simulink model "Python_Testing_Platform_2a"  (R2020b)
settings: Solver=VariableStepAuto  StartTime=0.0  StopTime=10.0  RelTol=1e-3
InitFcn:
  | close all
  | clear
  | clc
  | 
  | dtsim = 0.1;
  | dt =0.005;
  | dtdata = 0.01;
  | dtcontrol = 0.01;
  | 
  | % Enviromental Constants/System Parameters
  | 
  | mu = 398600; %km^3/s^2 (Earth)
  | 
  | I = [1.01560749 0.00028915 0.00002257;
  |        0.00028915 0.17343628 0.00936307;
  |        0.00002257 0.00936307 1.01561864];
  | 
  | I_inv =[1/I(1,1) 0 0; 0 1/I(2,2) 0; 0 0 1/I(3,3)];
  | 
  | % Inital Conditions
  | 
  | Y = 0;
  | P = 0;
  | R = 0;
  | 
  | a = 6378;
  | n = sqrt(mu/a^3);
  | 
  | wo = [0;0;0];
  | ho = [0;0;0];
  | 
  | % YPR to Quaternion
  | 
  | qo = [-cos(R/2)*sin(P/2)*sin(Y/2) + sin(R/2)*cos(P/2)*cos(Y/2);
  |           cos(R/2)*sin(P/2)*cos(Y/2) + sin(R/2)*cos(P/2)*sin(Y/2);
  |          -sin(R/2)*sin(P/2)*cos(Y/2) + cos(R/2)*cos(P/2)*sin(Y/2);
  |           sin(R/2)*sin(P/2)*sin(Y/2) + cos(R/2)*cos(P/2)*cos(Y/2)];
  | 
  | % Reaction Wheels
  | 
  | largeAngle = cosd(70);
  | smallAngle = sind(70);
  | e1 = [largeAngle; smallAngle; 0];
  | e2 = [largeAngle; 0; smallAngle];
  | e3 = [largeAngle; -smallAngle; 0];
  | e4 = [largeAngle; 0; -smallAngle];
  | e = [e1 e2 e3 e4];
  | 
  | % Reaction Wheels MOI and Ang Vel
  | 
  | Irw = 0.000453158;
  | 
  | w1 =1500*2*pi/60;
  | w2 = 1500*2*pi/60;
  | w3 = -1500*2*pi/60;
  | w4 = -1500*2*pi/60;
  | 
  | alpha_max = 1537.9; %rad/sec^2 Look at picture
  | 
  | Tmax = Irw*alpha_max; % Irw*alpha_max;
  | 
  | %User Input
  | 
  | Yt = 90*pi/180;
  | Pt = 10*pi/180;
  | Rt = 30*pi/180;
  | 
  | YPRtarget = [Yt, Pt, Rt];
  | 
  | %User Input Check
  | 
  | if Pt > 20*pi/180
  | 
  | error('Input a pitch angle lower that 20 degrees')
  | 
  | end
  | 
  | q_target = [-cos(Rt/2)*sin(Pt/2)*sin(Yt/2) + sin(Rt/2)*cos(Pt/2)*cos(Yt/2);
  |                   cos(Rt/2)*sin(Pt/2)*cos(Yt/2) + sin(Rt/2)*cos(Pt/2)*sin(Yt/2);
  |                  -sin(Rt/2)*sin(Pt/2)*cos(Yt/2) + cos(Rt/2)*cos(Pt/2)*sin(Yt/2);
  |                   sin(Rt/2)*sin(Pt/2)*sin(Yt/2) + cos(Rt/2)*cos(Pt/2)*cos(Yt/2)];
  | 
  | %LQR Controller
  | 
  | k1 = (I(2,2) - I(3,3))/I(1,1);
  | k2 = (I(2,2) - I(3,3))/I(2,2);
  | k3 = (I(2,2) - I(1,1))/I(3,3);
  | 
  | F = -2*n^2*[4*k1, 0, 0;0, 3*k2, 0; 0, 0, k3];
  | G = n*[0 0 (1-k1);0 0 0;(k3-1) 0 0 ];
  | 
  | A = [zeros(3,3) 0.5*eye(3);F G];
  | B = [zeros(3,3); I_inv];
  | R = eye(3);
  | R_inv = R^-1;
  | 
  | Q_nominal= diag([1,1,1,10,10,10]);
  | S_nominal = icare(A,B,Q_nominal,R);
  | K_nominal = -R_inv*B'*S_nominal;
  | 
  | Q_corrective= diag([1,1,1,10,10,10]);
  | S_corrective = icare(A,B,Q_corrective,R);
  | K_corrective = -R_inv*B'*S_corrective;
  | 
  | Q_yawsweep= diag([1,1,1,10,15,10]);
  | S_yawsweep = icare(A,B,Q_yawsweep,R);
  | K_yawsweep = -R_inv*B'*S_yawsweep;
libraries: dspinverses x1
settings Model: Creator=Eric Malmquist  LastModifiedBy=Eric Malmquist

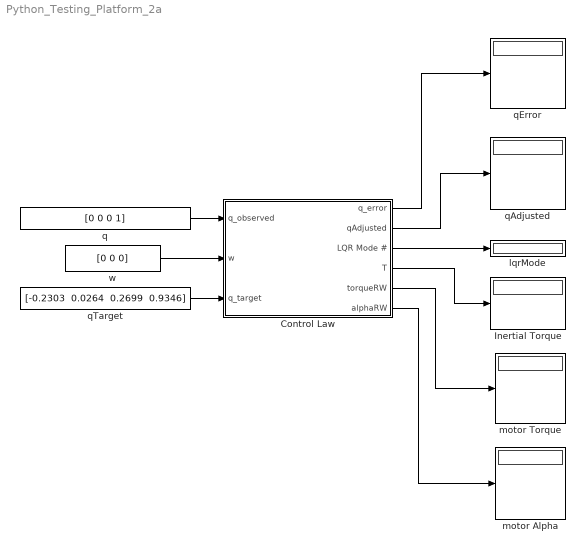
== system Python_Testing_Platform_2a ==
  Control Law : Subsystem
  Inertial Torque : Display
  lqrMode : Display
  motor Alpha : Display
  motor Torque : Display
  q : Constant  Value=[0 0 0 1]
  qAdjusted : Display
  qError : Display
  qTarget : Constant  Value="[-0.2303  0.0264  0.2699  0.9346]"
  w : Constant  Value=[0 0 0]
  wires:
  Control Law/4(T) -> Inertial Torque/1
  Control Law/2(qAdjusted) -> qAdjusted/1
  Control Law/3(LQR Mode #) -> lqrMode/1
  qTarget/1 -> Control Law/3(q_target)
  w/1 -> Control Law/2(w)
  Control Law/1(q_error) -> qError/1
  Control Law/5(torqueRW) -> motor Torque/1
  Control Law/6(alphaRW) -> motor Alpha/1
  q/1 -> Control Law/1(q_observed)

== system Python_Testing_Platform_2a/Control Law ==
  q_observed : Inport
  w : Inport  Port=2
  q_target : Inport  Port=3
  Controller1 : Subsystem
  Motor Control1 : Subsystem
  qerror1 : Subsystem
  q_error : Outport
  qAdjusted : Outport  Port=2
  LQR Mode # : Outport  Port=3
  T : Outport  Port=4
  torqueRW : Outport  Port=5
  alphaRW : Outport  Port=6
  wires:
  qerror1/3(Roll_ErrorAbs) -> Controller1/3(Roll_ErrorAbs)
  q_target/1 -> qerror1/1(q_target), Controller1/6(target)
  Controller1/3(Out1) -> LQR Mode #/1
  q_observed/1 -> qerror1/2(q_observed), Controller1/4(q_obs)
  Controller1/1(T) -> T/1, Motor Control1/1(T)
  qerror1/2(Yaw_ErrorAbs) -> Controller1/2(Yaw_ErrorAbs)
  qerror1/1(q_error) -> q_error/1, Controller1/1(q_error)
  w/1 -> Controller1/5(w)
  Motor Control1/1(torqueRW) -> torqueRW/1
  Motor Control1/2(alphaRW) -> alphaRW/1
  Controller1/2(qAdjusted) -> qAdjusted/1

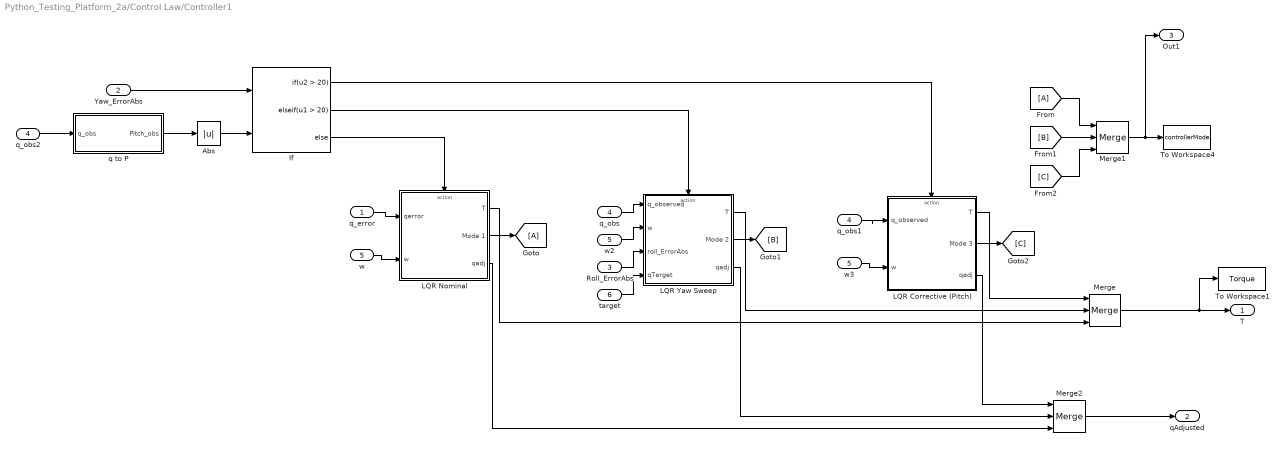
== system Python_Testing_Platform_2a/Control Law/Controller1 ==
  q_error : Inport
  Yaw_ErrorAbs : Inport  Port=2
  Roll_ErrorAbs : Inport  Port=3
  q_obs : Inport  Port=4
  w : Inport  Port=5
  target : Inport  Port=6
  Abs : Abs
  If : If  NumInputs=2  IfExpression=u2 > 20  ElseIfExpressions=u1 > 20
  LQR Corrective (Pitch) : Subsystem
  LQR Nominal : Subsystem  TreatAsAtomicUnit=on
  LQR Yaw Sweep : Subsystem
  Merge : Merge  Inputs=3
  Merge1 : Merge  Inputs=3
  Merge2 : Merge  Inputs=3
  To Workspace1 : ToWorkspace  VariableName=Torque  SaveFormat=Structure With Time  SampleTime=-1
  To Workspace4 : ToWorkspace  VariableName=controllerMode  SaveFormat=Structure With Time  SampleTime=-1
  q to P : Subsystem
  q_obs1 : InportShadow  Port=4
  q_obs2 : InportShadow  Port=4
  w2 : InportShadow  Port=5
  w3 : InportShadow  Port=5
  T : Outport
  qAdjusted : Outport  Port=2
  Out1 : Outport  Port=3
  wires:
  Yaw_ErrorAbs/1 -> If/1
  If/3 -> LQR Nominal/Action
  q_error/1 -> LQR Nominal/1(qerror)
  If/1 -> LQR Corrective (Pitch)/Action
  q_obs1/1 -> LQR Corrective (Pitch)/1(q_observed)
  q_obs/1 -> LQR Yaw Sweep/1(q_observed)
  q to P/1(Pitch_obs) -> Abs/1
  If/2 -> LQR Yaw Sweep/Action
  LQR Nominal/2(Mode 1) -> [A]
  LQR Yaw Sweep/2(Mode 2) -> [B]
  LQR Corrective (Pitch)/2(Mode 3) -> [C]
  [B] -> Merge1/2
  [A] -> Merge1/1
  [C] -> Merge1/3
  Merge1/1 -> Out1/1, To Workspace4/1
  w3/1 -> LQR Corrective (Pitch)/2(w)
  w2/1 -> LQR Yaw Sweep/2(w)
  w/1 -> LQR Nominal/2(w)
  q_obs2/1 -> q to P/1(q_obs)
  Abs/1 -> If/2
  Roll_ErrorAbs/1 -> LQR Yaw Sweep/3(roll_ErrorAbs)
  LQR Nominal/1(T) -> Merge/3
  LQR Yaw Sweep/1(T) -> Merge/2
  LQR Corrective (Pitch)/1(T) -> Merge/1
  Merge/1 -> To Workspace1/1, T/1
  LQR Nominal/3(qadj) -> Merge2/3
  LQR Yaw Sweep/3(qadj) -> Merge2/2
  LQR Corrective (Pitch)/3(qadj) -> Merge2/1
  Merge2/1 -> qAdjusted/1
  target/1 -> LQR Yaw Sweep/4(qTarget)

== system Python_Testing_Platform_2a/Control Law/Motor Control1 ==
  T : Inport
  Actuator : Subsystem
  torqueRW : Outport
  alphaRW : Outport  Port=2
  wires:
  T/1 -> Actuator/1(Torque)
  Actuator/2(torque) -> torqueRW/1
  Actuator/1(alpha_RW) -> alphaRW/1

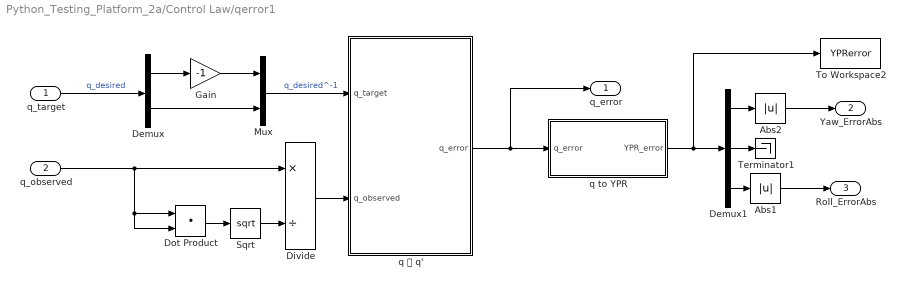
== system Python_Testing_Platform_2a/Control Law/qerror1 ==
  q_target : Inport
  q_observed : Inport  Port=2
  Abs1 : Abs
  Abs2 : Abs
  Demux : Demux  Outputs=[3,1]
  Demux1 : Demux  Outputs=3
  Divide : Product  Inputs=*/
  Dot Product : DotProduct  InputSameDT=on  OutDataTypeStr=Inherit: Inherit via internal rule
  Gain : Gain  Gain=-1
  Mux : Mux  Inputs=2
  Sqrt : Sqrt  SaturateOnIntegerOverflow=on
  Terminator1 : Terminator
  To Workspace2 : ToWorkspace  VariableName=YPRerror  SaveFormat=Structure With Time  SampleTime=-1
  q to YPR : Subsystem  TreatAsAtomicUnit=on
  q ⦻ q' : Subsystem  TreatAsAtomicUnit=on
  q_error : Outport
  Yaw_ErrorAbs : Outport  Port=2
  Roll_ErrorAbs : Outport  Port=3
  wires:
  Abs2/1 -> Yaw_ErrorAbs/1
  Demux1/2 -> Terminator1/1
  Abs1/1 -> Roll_ErrorAbs/1
  Divide/1 -> q ⦻ q'/2(q_observed)
  q_observed/1 -> Divide/1, Dot Product/1, Dot Product/2
  Dot Product/1 -> Sqrt/1
  q ⦻ q'/1(q_error) -> q to YPR/1(q_error), q_error/1
  Gain/1 -> Mux/1
  Mux/1 -> q ⦻ q'/1(q_target)  "q_desired^-1"
  q_target/1 -> Demux/1  "q_desired"
  Demux/1 -> Gain/1
  Sqrt/1 -> Divide/2
  Demux/2 -> Mux/2
  q to YPR/1(YPR_error) -> Demux1/1, To Workspace2/1
  Demux1/1 -> Abs2/1
  Demux1/3 -> Abs1/1

== system Python_Testing_Platform_2a/Control Law/Controller1/LQR Corrective (Pitch) ==
  q_observed : Inport
  w : Inport  Port=2
  Action Port : ActionPort  ActionPortLabel=if(u2 > 20)
  Constant : Constant  Value=3
  LQR Corrective (Pitch) : Subsystem
  q_adjustment : Subsystem
  q_error : Subsystem
  T : Outport
  Mode 3 : Outport  Port=2
  qadj : Outport  Port=3
  wires:
  Constant/1 -> Mode 3/1
  LQR Corrective (Pitch)/1(T) -> T/1
  w/1 -> LQR Corrective (Pitch)/2(w)
  q_adjustment/1(q_adjusted) -> q_error/1(q_target)
  q_observed/1 -> q_adjustment/1(q_obs), q_error/2(q_observed)
  q_error/1(q_error) -> qadj/1, LQR Corrective (Pitch)/1(q_error)

== system Python_Testing_Platform_2a/Control Law/Controller1/LQR Nominal ==
  qerror : Inport
  w : Inport  Port=2
  Action Port : ActionPort  ActionPortLabel=else
  Constant : Constant
  LQR Nominal : Subsystem
  T : Outport
  Mode 1 : Outport  Port=2
  qadj : Outport  Port=3
  wires:
  Constant/1 -> Mode 1/1
  LQR Nominal/1(T) -> T/1
  w/1 -> LQR Nominal/2(w)
  qerror/1 -> qadj/1, LQR Nominal/1(q_error)

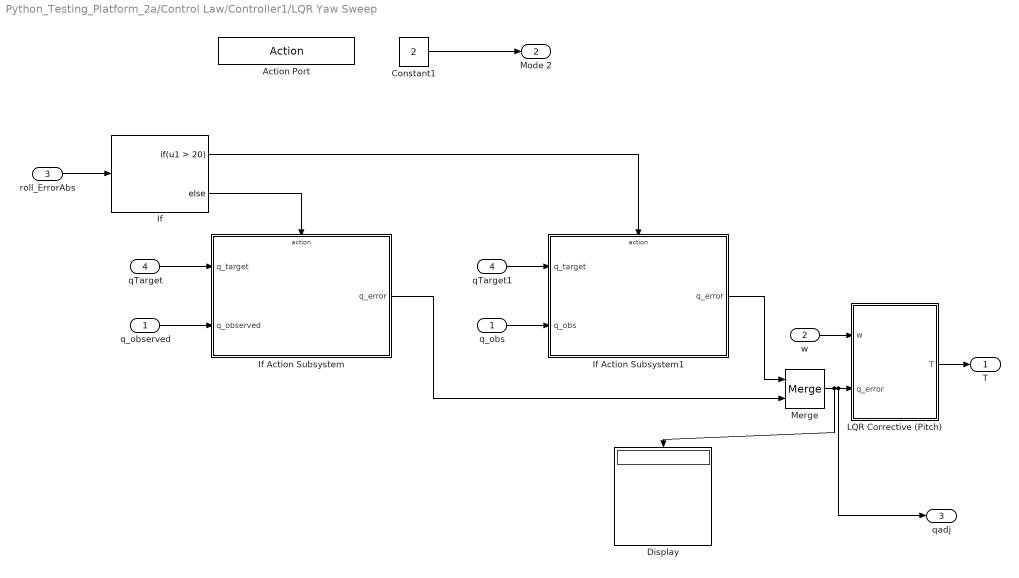
== system Python_Testing_Platform_2a/Control Law/Controller1/LQR Yaw Sweep ==
  q_observed : Inport
  w : Inport  Port=2
  roll_ErrorAbs : Inport  Port=3
  qTarget : Inport  Port=4
  Action Port : ActionPort  ActionPortLabel=elseif(u1 > 20)
  Constant1 : Constant  Value=2
  Display : Display
  If : If  IfExpression=u1 > 20
  If Action Subsystem : Subsystem  TreatAsAtomicUnit=on
  If Action Subsystem1 : Subsystem  TreatAsAtomicUnit=on
  LQR Corrective (Pitch) : Subsystem
  Merge : Merge
  qTarget1 : InportShadow  Port=4
  q_obs : InportShadow
  T : Outport
  Mode 2 : Outport  Port=2
  qadj : Outport  Port=3
  wires:
  roll_ErrorAbs/1 -> If/1
  qTarget/1 -> If Action Subsystem/1(q_target)
  Constant1/1 -> Mode 2/1
  If/2 -> If Action Subsystem/Action
  LQR Corrective (Pitch)/1(T) -> T/1
  w/1 -> LQR Corrective (Pitch)/1(w)
  If/1 -> If Action Subsystem1/Action
  q_observed/1 -> If Action Subsystem/2(q_observed)
  Merge/1 -> Display/1, qadj/1, LQR Corrective (Pitch)/2(q_error)
  If Action Subsystem1/1(q_error) -> Merge/1
  If Action Subsystem/1(q_error) -> Merge/2
  q_obs/1 -> If Action Subsystem1/2(q_obs)
  qTarget1/1 -> If Action Subsystem1/1(q_target)

== system Python_Testing_Platform_2a/Control Law/Controller1/q to P ==
  q_obs : Inport
  -DCM(1,3) : Fcn  Expr=-2*(u(1)*u(3) - u(2)*u(4))
  Gain2 : Gain  Gain=180/pi
  Trigonometric Function1 : Trigonometry  Operator=asin
  Pitch_obs : Outport
  wires:
  Gain2/1 -> Pitch_obs/1
  Trigonometric Function1/1 -> Gain2/1  "P"
  -DCM(1,3)/1 -> Trigonometric Function1/1
  q_obs/1 -> -DCM(1,3)/1

== system Python_Testing_Platform_2a/Control Law/Motor Control1/Actuator ==
  Torque : Inport  PortDimensions=[3,1]
  Constant1 : Constant  Value=Irw
  Constant2 : Constant  Value=e
  Constant3 : Constant  Value=Irw
  Gain : Gain  Gain=-1
  Multiply : Product  Multiplication=Matrix(*)
  Product : Product
  Product1 : Product
  Pseudoinverse : dspinverses/Pseudoinverse  wanterr=off  SimulateUsing=Interpreted execution
      settings: SourceProductBaseCode=DS
  Rate Transition1 : RateTransition  InitialCondition=[0;0;0;0]  OutPortSampleTime=dtdata
  alpha_RW : Outport
  torque : Outport  Port=2
  wires:
  Torque/1 -> Gain/1
  Product/1 -> Pseudoinverse/1
  Constant1/1 -> Product/1
  Pseudoinverse/1 -> Multiply/1  "psiv(A)"
  Multiply/1 -> Product1/1, alpha_RW/1  "alpha_RW"
  Constant2/1 -> Product/2  "A"
  Gain/1 -> Multiply/2
  Constant3/1 -> Product1/2
  Product1/1 -> Rate Transition1/1
  Rate Transition1/1 -> torque/1

== system Python_Testing_Platform_2a/Control Law/qerror1/q to YPR ==
  note: Quaternion to Euler Angles using sequency 3-2-1
  q_error : Inport
  -DCM(1,3) : Fcn  Expr=-2*(u(1)*u(3) - u(2)*u(4))
  DCM(1,1) : Fcn  Expr=u(4)^2 + u(1)^2 - u(2)^2 - u(3)^2
  DCM(1,2) : Fcn  Expr=2*(u(1)*u(2) + u(3)*u(4))
  DCM(2,3) : Fcn  Expr=2*(u(2)*u(3) + u(1)*u(4))
  DCM(3,3) : Fcn  Expr=u(4)^2 - u(1)^2 - u(2)^2 + u(3)^2
  Gain2 : Gain  Gain=180/pi
  Mux : Mux  Inputs=3
  Trigonometric Function : Trigonometry  Operator=asin
  Trigonometric Function1 : Trigonometry  Operator=atan2
  Trigonometric Function2 : Trigonometry  Operator=atan2
  YPR_error : Outport
  wires:
  q_error/1 -> DCM(3,3)/1, DCM(2,3)/1, -DCM(1,3)/1, DCM(1,2)/1, DCM(1,1)/1
  -DCM(1,3)/1 -> Trigonometric Function/1
  DCM(2,3)/1 -> Trigonometric Function2/1
  DCM(1,2)/1 -> Trigonometric Function1/1
  DCM(1,1)/1 -> Trigonometric Function1/2
  DCM(3,3)/1 -> Trigonometric Function2/2
  Trigonometric Function/1 -> Mux/2  "P"
  Trigonometric Function2/1 -> Mux/3  "R"
  Trigonometric Function1/1 -> Mux/1  "Y"
  Gain2/1 -> YPR_error/1
  Mux/1 -> Gain2/1

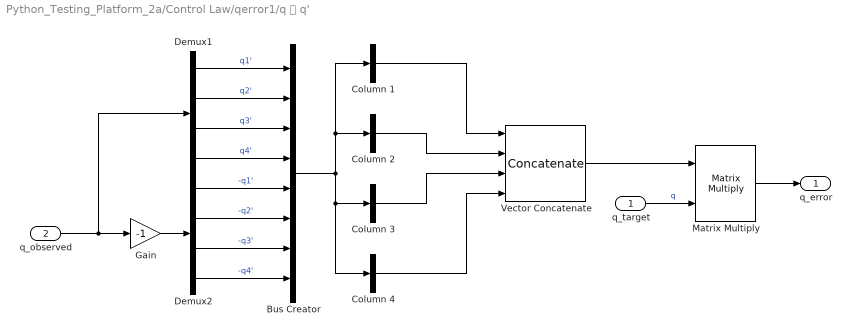
== system Python_Testing_Platform_2a/Control Law/qerror1/q ⦻ q' ==
  q_target : Inport
  q_observed : Inport  Port=2
  Bus Creator : BusCreator  Inputs=8
  Column 1 : BusSelector  OutputSignals=q4',-q3',q2',-q1'  OutputAsBus=on
  Column 2 : BusSelector  OutputSignals=q3',q4',-q1',-q2'  OutputAsBus=on
  Column 3 : BusSelector  OutputSignals=-q2',q1',q4',-q3'  OutputAsBus=on
  Column 4 : BusSelector  OutputSignals=q1',q2',q3',q4'  OutputAsBus=on
  Demux1 : Demux
  Demux2 : Demux
  Gain : Gain  Gain=-1
  Matrix Multiply : Product  Multiplication=Matrix(*)
  Vector Concatenate : Concatenate  NumInputs=4  Mode=Multidimensional array  ConcatenateDimension=2
  q_error : Outport
  wires:
  Gain/1 -> Demux2/1
  Demux1/1 -> Bus Creator/1  "q1'"
  Demux1/3 -> Bus Creator/3  "q3'"
  Demux1/2 -> Bus Creator/2  "q2'"
  Demux2/4 -> Bus Creator/8  "-q4'"
  Demux2/3 -> Bus Creator/7  "-q3'"
  Demux2/2 -> Bus Creator/6  "-q2'"
  Demux2/1 -> Bus Creator/5  "-q1'"
  Demux1/4 -> Bus Creator/4  "q4'"
  Bus Creator/1 -> Column 4/1, Column 3/1, Column 1/1, Column 2/1
  Column 1/1 -> Vector Concatenate/1
  Column 2/1 -> Vector Concatenate/2
  Column 3/1 -> Vector Concatenate/3
  Column 4/1 -> Vector Concatenate/4
  q_observed/1 -> Demux1/1, Gain/1
  q_target/1 -> Matrix Multiply/2  "q"
  Matrix Multiply/1 -> q_error/1
  Vector Concatenate/1 -> Matrix Multiply/1

== system Python_Testing_Platform_2a/Control Law/Controller1/LQR Corrective (Pitch)/LQR Corrective (Pitch) ==
  q_error : Inport
  w : Inport  Port=2
  Constant3 : Constant  Value=K_corrective
  Demux1 : Demux  Outputs=[3,1]
  Mux1 : Mux  Inputs=2
  Product : Product  Multiplication=Matrix(*)
  Terminator1 : Terminator
  T : Outport
  wires:
  Product/1 -> T/1
  q_error/1 -> Demux1/1
  Constant3/1 -> Product/1
  Demux1/1 -> Mux1/1  "qhat_Error"
  w/1 -> Mux1/2
  Mux1/1 -> Product/2  "xbar"
  Demux1/2 -> Terminator1/1

== system Python_Testing_Platform_2a/Control Law/Controller1/LQR Corrective (Pitch)/q_adjustment ==
  q_obs : Inport
  DCM(1,1) : Fcn  Expr=u(4)^2 + u(1)^2 - u(2)^2 - u(3)^2
  DCM(1,2) : Fcn  Expr=2*(u(1)*u(2) + u(3)*u(4))
  DCM(2,3) : Fcn  Expr=2*(u(2)*u(3) + u(1)*u(4))
  DCM(3,3) : Fcn  Expr=u(4)^2 - u(1)^2 - u(2)^2 + u(3)^2
  Trigonometric Function4 : Trigonometry  Operator=atan2
  Trigonometric Function5 : Trigonometry  Operator=atan2
  YPR to q : Subsystem
  q_adjusted : Outport
  wires:
  Trigonometric Function5/1 -> YPR to q/2(R)  "R"
  DCM(2,3)/1 -> Trigonometric Function5/1
  DCM(1,1)/1 -> Trigonometric Function4/2
  DCM(3,3)/1 -> Trigonometric Function5/2
  DCM(1,2)/1 -> Trigonometric Function4/1
  q_obs/1 -> DCM(3,3)/1, DCM(2,3)/1, DCM(1,2)/1, DCM(1,1)/1
  YPR to q/1(q_adjusted) -> q_adjusted/1
  Trigonometric Function4/1 -> YPR to q/1(Y)  "Y"

== system Python_Testing_Platform_2a/Control Law/Controller1/LQR Corrective (Pitch)/q_error ==
  q_target : Inport
  q_observed : Inport  Port=2
  Demux : Demux  Outputs=[3,1]
  Divide : Product  Inputs=*/
  Dot Product : DotProduct  InputSameDT=on  OutDataTypeStr=Inherit: Inherit via internal rule
  Gain : Gain  Gain=-1
  Mux : Mux  Inputs=2
  Sqrt : Sqrt  SaturateOnIntegerOverflow=on
  q ⦻ q' : Subsystem  TreatAsAtomicUnit=on
  q_error : Outport
  wires:
  q ⦻ q'/1(q_error) -> q_error/1
  Mux/1 -> q ⦻ q'/1(q_target)  "q_desired^-1"
  Sqrt/1 -> Divide/2
  Demux/1 -> Gain/1
  q_target/1 -> Demux/1  "q_desired"
  Gain/1 -> Mux/1
  q_observed/1 -> Divide/1, Dot Product/1, Dot Product/2
  Dot Product/1 -> Sqrt/1
  Demux/2 -> Mux/2
  Divide/1 -> q ⦻ q'/2(q_observed)

== system Python_Testing_Platform_2a/Control Law/Controller1/LQR Nominal/LQR Nominal ==
  q_error : Inport
  w : Inport  Port=2
  Constant3 : Constant  Value=K_nominal
  Demux1 : Demux  Outputs=[3,1]
  Mux1 : Mux  Inputs=2
  Product : Product  Multiplication=Matrix(*)
  Terminator1 : Terminator
  T : Outport
  wires:
  Mux1/1 -> Product/2  "xbar"
  Demux1/1 -> Mux1/1  "qhat_Error"
  q_error/1 -> Demux1/1
  Demux1/2 -> Terminator1/1
  w/1 -> Mux1/2
  Constant3/1 -> Product/1
  Product/1 -> T/1

== system Python_Testing_Platform_2a/Control Law/Controller1/LQR Yaw Sweep/If Action Subsystem ==
  q_target : Inport
  q_observed : Inport  Port=2
  Action Port : ActionPort  ActionPortLabel=else
  Display : Display
  Display1 : Display
  Display2 : Display
  q_adjustment : Subsystem
  qerror : Subsystem
  q_error : Outport
  wires:
  q_target/1 -> q_adjustment/1(q_target), Display2/1
  qerror/1(q_error) -> Display1/1, q_error/1
  q_observed/1 -> Display/1, qerror/2(q_observed)
  q_adjustment/1(q_adjusted) -> qerror/1(q_target)

== system Python_Testing_Platform_2a/Control Law/Controller1/LQR Yaw Sweep/If Action Subsystem1 ==
  q_target : Inport
  q_obs : Inport  Port=2
  Action Port : ActionPort  ActionPortLabel=if(u1 > 20)
  q_adjustment : Subsystem
  qerror : Subsystem
  q_error : Outport
  wires:
  q_adjustment/1(q_adjusted) -> qerror/1(q_target)
  q_target/1 -> q_adjustment/1(q_target)
  q_obs/1 -> qerror/2(q_observed), q_adjustment/2(q_obs)
  qerror/1(q_error) -> q_error/1

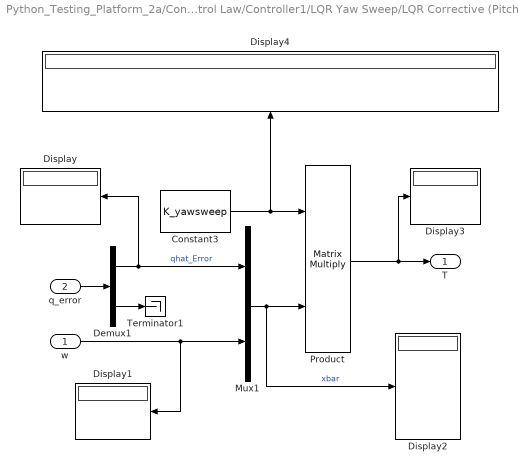
== system Python_Testing_Platform_2a/Control Law/Controller1/LQR Yaw Sweep/LQR Corrective (Pitch) ==
  w : Inport
  q_error : Inport  Port=2
  Constant3 : Constant  Value=K_yawsweep
  Demux1 : Demux  Outputs=[3,1]
  Display{,1..4} (5 alike) : Display
  Mux1 : Mux  Inputs=2
  Product : Product  Multiplication=Matrix(*)
  Terminator1 : Terminator
  T : Outport
  wires:
  Product/1 -> Display3/1, T/1
  q_error/1 -> Demux1/1
  Constant3/1 -> Product/1, Display4/1
  Demux1/1 -> Display/1, Mux1/1  "qhat_Error"
  w/1 -> Display1/1, Mux1/2
  Mux1/1 -> Display2/1, Product/2  "xbar"
  Demux1/2 -> Terminator1/1

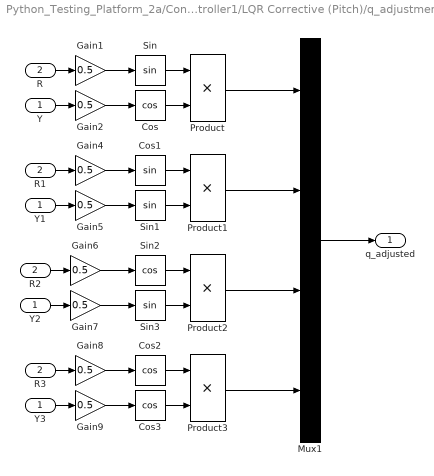
== system Python_Testing_Platform_2a/Control Law/Controller1/LQR Corrective (Pitch)/q_adjustment/YPR to q ==
  Y : Inport
  R : Inport  Port=2
  Cos : Trigonometry  Operator=cos
  Cos1 : Trigonometry
  Cos2 : Trigonometry  Operator=cos
  Cos3 : Trigonometry  Operator=cos
  Gain{1..2,4..9} (8 alike) : Gain  Gain=0.5
  Mux1 : Mux
  Product{,1..3} (4 alike) : Product
  R1 : InportShadow  Port=2
  R2 : InportShadow  Port=2
  R3 : InportShadow  Port=2
  Sin : Trigonometry
  Sin1 : Trigonometry
  Sin2 : Trigonometry  Operator=cos
  Sin3 : Trigonometry
  Y1 : InportShadow
  Y2 : InportShadow
  Y3 : InportShadow
  q_adjusted : Outport
  wires:
  Gain2/1 -> Cos/1
  Sin/1 -> Product/1
  Sin3/1 -> Product2/2
  Sin1/1 -> Product1/2
  Mux1/1 -> q_adjusted/1
  Cos/1 -> Product/2
  Sin2/1 -> Product2/1
  Gain8/1 -> Cos2/1
  Cos1/1 -> Product1/1
  Gain6/1 -> Sin2/1
  Product3/1 -> Mux1/4
  Product/1 -> Mux1/1
  Gain5/1 -> Sin1/1
  Gain9/1 -> Cos3/1
  Gain4/1 -> Cos1/1
  Cos2/1 -> Product3/1
  Product1/1 -> Mux1/2
  Gain7/1 -> Sin3/1
  Gain1/1 -> Sin/1
  Cos3/1 -> Product3/2
  R1/1 -> Gain4/1
  Y1/1 -> Gain5/1
  R2/1 -> Gain6/1
  Y2/1 -> Gain7/1
  Y3/1 -> Gain9/1
  R3/1 -> Gain8/1
  Y/1 -> Gain2/1
  R/1 -> Gain1/1
  Product2/1 -> Mux1/3

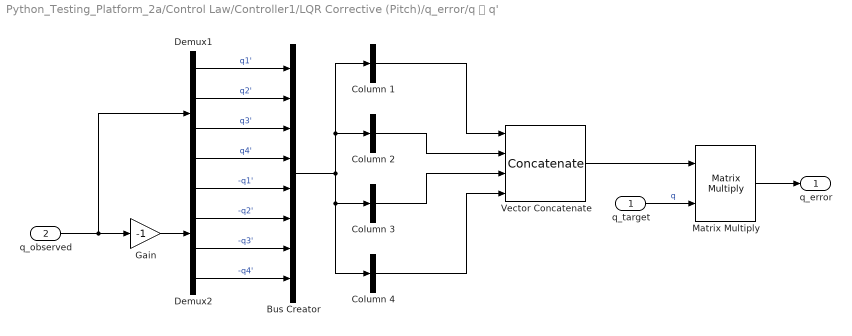
== system Python_Testing_Platform_2a/Control Law/Controller1/LQR Corrective (Pitch)/q_error/q ⦻ q' ==
  q_target : Inport
  q_observed : Inport  Port=2
  Bus Creator : BusCreator  Inputs=8
  Column 1 : BusSelector  OutputSignals=q4',-q3',q2',-q1'  OutputAsBus=on
  Column 2 : BusSelector  OutputSignals=q3',q4',-q1',-q2'  OutputAsBus=on
  Column 3 : BusSelector  OutputSignals=-q2',q1',q4',-q3'  OutputAsBus=on
  Column 4 : BusSelector  OutputSignals=q1',q2',q3',q4'  OutputAsBus=on
  Demux1 : Demux
  Demux2 : Demux
  Gain : Gain  Gain=-1
  Matrix Multiply : Product  Multiplication=Matrix(*)
  Vector Concatenate : Concatenate  NumInputs=4  Mode=Multidimensional array  ConcatenateDimension=2
  q_error : Outport
  wires:
  Gain/1 -> Demux2/1
  Demux1/1 -> Bus Creator/1  "q1'"
  Demux1/3 -> Bus Creator/3  "q3'"
  Demux1/2 -> Bus Creator/2  "q2'"
  Demux2/4 -> Bus Creator/8  "-q4'"
  Demux2/3 -> Bus Creator/7  "-q3'"
  Demux2/2 -> Bus Creator/6  "-q2'"
  Demux2/1 -> Bus Creator/5  "-q1'"
  Demux1/4 -> Bus Creator/4  "q4'"
  Bus Creator/1 -> Column 4/1, Column 3/1, Column 1/1, Column 2/1
  Column 1/1 -> Vector Concatenate/1
  Column 2/1 -> Vector Concatenate/2
  Column 3/1 -> Vector Concatenate/3
  Column 4/1 -> Vector Concatenate/4
  q_observed/1 -> Demux1/1, Gain/1
  q_target/1 -> Matrix Multiply/2  "q"
  Matrix Multiply/1 -> q_error/1
  Vector Concatenate/1 -> Matrix Multiply/1

== system Python_Testing_Platform_2a/Control Law/Controller1/LQR Yaw Sweep/If Action Subsystem/q_adjustment ==
  q_target : Inport
  DCM(1,1) : Fcn  Expr=u(4)^2 + u(1)^2 - u(2)^2 - u(3)^2
  DCM(1,2) : Fcn  Expr=2*(u(1)*u(2) + u(3)*u(4))
  DCM(2,3) : Fcn  Expr=2*(u(2)*u(3) + u(1)*u(4))
  DCM(3,3) : Fcn  Expr=u(4)^2 - u(1)^2 - u(2)^2 + u(3)^2
  Trigonometric Function4 : Trigonometry  Operator=atan2
  Trigonometric Function5 : Trigonometry  Operator=atan2
  YPR to q : Subsystem
  q_adjusted : Outport
  wires:
  YPR to q/1(q_adjusted) -> q_adjusted/1
  Trigonometric Function5/1 -> YPR to q/2(R)  "R"
  DCM(3,3)/1 -> Trigonometric Function5/2
  DCM(1,1)/1 -> Trigonometric Function4/2
  DCM(2,3)/1 -> Trigonometric Function5/1
  Trigonometric Function4/1 -> YPR to q/1(Y)  "Y"
  DCM(1,2)/1 -> Trigonometric Function4/1
  q_target/1 -> DCM(3,3)/1, DCM(2,3)/1, DCM(1,2)/1, DCM(1,1)/1

== system Python_Testing_Platform_2a/Control Law/Controller1/LQR Yaw Sweep/If Action Subsystem/qerror ==
  q_target : Inport
  q_observed : Inport  Port=2
  Demux : Demux  Outputs=[3,1]
  Divide : Product  Inputs=*/
  Dot Product : DotProduct  InputSameDT=on  OutDataTypeStr=Inherit: Inherit via internal rule
  Gain : Gain  Gain=-1
  Mux : Mux  Inputs=2
  Sqrt : Sqrt  SaturateOnIntegerOverflow=on
  q ⦻ q' : Subsystem  TreatAsAtomicUnit=on
  q_error : Outport
  wires:
  Sqrt/1 -> Divide/2
  Dot Product/1 -> Sqrt/1
  Gain/1 -> Mux/1
  Mux/1 -> q ⦻ q'/1(q_target)  "q_desired^-1"
  q ⦻ q'/1(q_error) -> q_error/1
  q_observed/1 -> Divide/1, Dot Product/1, Dot Product/2
  q_target/1 -> Demux/1  "q_desired"
  Demux/1 -> Gain/1
  Demux/2 -> Mux/2
  Divide/1 -> q ⦻ q'/2(q_observed)

== system Python_Testing_Platform_2a/Control Law/Controller1/LQR Yaw Sweep/If Action Subsystem1/q_adjustment ==
  q_target : Inport
  q_obs : Inport  Port=2
  DCM(1,1) : Fcn  Expr=u(4)^2 + u(1)^2 - u(2)^2 - u(3)^2
  DCM(1,2) : Fcn  Expr=2*(u(1)*u(2) + u(3)*u(4))
  DCM(2,3) : Fcn  Expr=2*(u(2)*u(3) + u(1)*u(4))
  DCM(3,3) : Fcn  Expr=u(4)^2 - u(1)^2 - u(2)^2 + u(3)^2
  Trigonometric Function4 : Trigonometry  Operator=atan2
  Trigonometric Function5 : Trigonometry  Operator=atan2
  YPR to q : Subsystem
  q_adjusted : Outport
  wires:
  YPR to q/1(q_adjusted) -> q_adjusted/1
  Trigonometric Function5/1 -> YPR to q/2(R)  "R"
  DCM(1,1)/1 -> Trigonometric Function4/2
  DCM(3,3)/1 -> Trigonometric Function5/2
  DCM(1,2)/1 -> Trigonometric Function4/1
  DCM(2,3)/1 -> Trigonometric Function5/1
  Trigonometric Function4/1 -> YPR to q/1(Y)  "Y"
  q_target/1 -> DCM(1,1)/1, DCM(1,2)/1
  q_obs/1 -> DCM(2,3)/1, DCM(3,3)/1

== system Python_Testing_Platform_2a/Control Law/Controller1/LQR Yaw Sweep/If Action Subsystem1/qerror ==
  q_target : Inport
  q_observed : Inport  Port=2
  Demux : Demux  Outputs=[3,1]
  Divide : Product  Inputs=*/
  Dot Product : DotProduct  InputSameDT=on  OutDataTypeStr=Inherit: Inherit via internal rule
  Gain : Gain  Gain=-1
  Mux : Mux  Inputs=2
  Sqrt : Sqrt  SaturateOnIntegerOverflow=on
  q ⦻ q' : Subsystem  TreatAsAtomicUnit=on
  q_error : Outport
  wires:
  q ⦻ q'/1(q_error) -> q_error/1
  Mux/1 -> q ⦻ q'/1(q_target)  "q_desired^-1"
  Sqrt/1 -> Divide/2
  Demux/1 -> Gain/1
  q_target/1 -> Demux/1  "q_desired"
  Gain/1 -> Mux/1
  q_observed/1 -> Divide/1, Dot Product/1, Dot Product/2
  Dot Product/1 -> Sqrt/1
  Demux/2 -> Mux/2
  Divide/1 -> q ⦻ q'/2(q_observed)

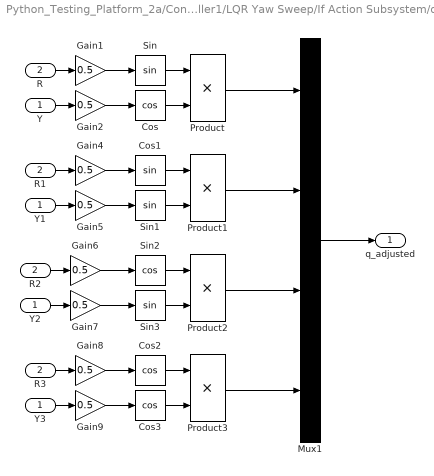
== system Python_Testing_Platform_2a/Control Law/Controller1/LQR Yaw Sweep/If Action Subsystem/q_adjustment/YPR to q ==
  Y : Inport
  R : Inport  Port=2
  Cos : Trigonometry  Operator=cos
  Cos1 : Trigonometry
  Cos2 : Trigonometry  Operator=cos
  Cos3 : Trigonometry  Operator=cos
  Gain{1..2,4..9} (8 alike) : Gain  Gain=0.5
  Mux1 : Mux
  Product{,1..3} (4 alike) : Product
  R1 : InportShadow  Port=2
  R2 : InportShadow  Port=2
  R3 : InportShadow  Port=2
  Sin : Trigonometry
  Sin1 : Trigonometry
  Sin2 : Trigonometry  Operator=cos
  Sin3 : Trigonometry
  Y1 : InportShadow
  Y2 : InportShadow
  Y3 : InportShadow
  q_adjusted : Outport
  wires:
  Gain2/1 -> Cos/1
  Sin/1 -> Product/1
  Sin3/1 -> Product2/2
  Sin1/1 -> Product1/2
  Mux1/1 -> q_adjusted/1
  Cos/1 -> Product/2
  Sin2/1 -> Product2/1
  Gain8/1 -> Cos2/1
  Cos1/1 -> Product1/1
  Gain6/1 -> Sin2/1
  Product3/1 -> Mux1/4
  Product/1 -> Mux1/1
  Gain5/1 -> Sin1/1
  Gain9/1 -> Cos3/1
  Gain4/1 -> Cos1/1
  Cos2/1 -> Product3/1
  Product1/1 -> Mux1/2
  Gain7/1 -> Sin3/1
  Gain1/1 -> Sin/1
  Cos3/1 -> Product3/2
  R1/1 -> Gain4/1
  Y1/1 -> Gain5/1
  R2/1 -> Gain6/1
  Y2/1 -> Gain7/1
  Y3/1 -> Gain9/1
  R3/1 -> Gain8/1
  Y/1 -> Gain2/1
  R/1 -> Gain1/1
  Product2/1 -> Mux1/3

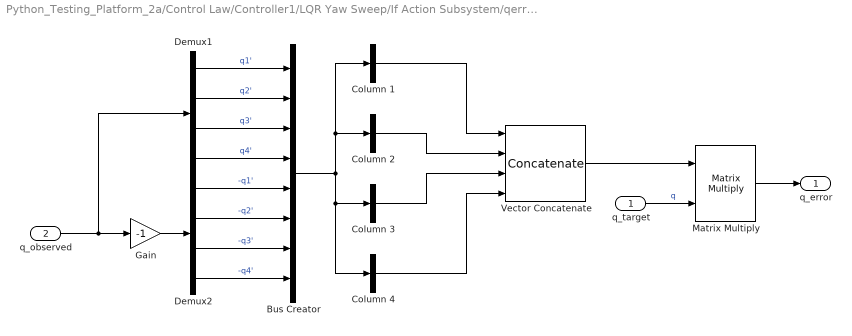
== system Python_Testing_Platform_2a/Control Law/Controller1/LQR Yaw Sweep/If Action Subsystem/qerror/q ⦻ q' ==
  q_target : Inport
  q_observed : Inport  Port=2
  Bus Creator : BusCreator  Inputs=8
  Column 1 : BusSelector  OutputSignals=q4',-q3',q2',-q1'  OutputAsBus=on
  Column 2 : BusSelector  OutputSignals=q3',q4',-q1',-q2'  OutputAsBus=on
  Column 3 : BusSelector  OutputSignals=-q2',q1',q4',-q3'  OutputAsBus=on
  Column 4 : BusSelector  OutputSignals=q1',q2',q3',q4'  OutputAsBus=on
  Demux1 : Demux
  Demux2 : Demux
  Gain : Gain  Gain=-1
  Matrix Multiply : Product  Multiplication=Matrix(*)
  Vector Concatenate : Concatenate  NumInputs=4  Mode=Multidimensional array  ConcatenateDimension=2
  q_error : Outport
  wires:
  Gain/1 -> Demux2/1
  Demux1/1 -> Bus Creator/1  "q1'"
  Demux1/3 -> Bus Creator/3  "q3'"
  Demux1/2 -> Bus Creator/2  "q2'"
  Demux2/4 -> Bus Creator/8  "-q4'"
  Demux2/3 -> Bus Creator/7  "-q3'"
  Demux2/2 -> Bus Creator/6  "-q2'"
  Demux2/1 -> Bus Creator/5  "-q1'"
  Demux1/4 -> Bus Creator/4  "q4'"
  Bus Creator/1 -> Column 4/1, Column 3/1, Column 1/1, Column 2/1
  Column 1/1 -> Vector Concatenate/1
  Column 2/1 -> Vector Concatenate/2
  Column 3/1 -> Vector Concatenate/3
  Column 4/1 -> Vector Concatenate/4
  q_observed/1 -> Demux1/1, Gain/1
  q_target/1 -> Matrix Multiply/2  "q"
  Matrix Multiply/1 -> q_error/1
  Vector Concatenate/1 -> Matrix Multiply/1

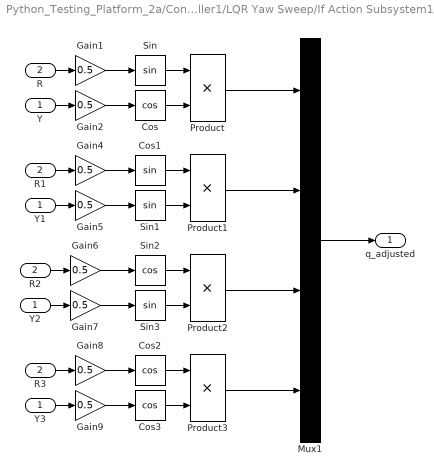
== system Python_Testing_Platform_2a/Control Law/Controller1/LQR Yaw Sweep/If Action Subsystem1/q_adjustment/YPR to q ==
  Y : Inport
  R : Inport  Port=2
  Cos : Trigonometry  Operator=cos
  Cos1 : Trigonometry
  Cos2 : Trigonometry  Operator=cos
  Cos3 : Trigonometry  Operator=cos
  Gain{1..2,4..9} (8 alike) : Gain  Gain=0.5
  Mux1 : Mux
  Product{,1..3} (4 alike) : Product
  R1 : InportShadow  Port=2
  R2 : InportShadow  Port=2
  R3 : InportShadow  Port=2
  Sin : Trigonometry
  Sin1 : Trigonometry
  Sin2 : Trigonometry  Operator=cos
  Sin3 : Trigonometry
  Y1 : InportShadow
  Y2 : InportShadow
  Y3 : InportShadow
  q_adjusted : Outport
  wires:
  Gain2/1 -> Cos/1
  Sin/1 -> Product/1
  Sin3/1 -> Product2/2
  Sin1/1 -> Product1/2
  Mux1/1 -> q_adjusted/1
  Cos/1 -> Product/2
  Sin2/1 -> Product2/1
  Gain8/1 -> Cos2/1
  Cos1/1 -> Product1/1
  Gain6/1 -> Sin2/1
  Product3/1 -> Mux1/4
  Product/1 -> Mux1/1
  Gain5/1 -> Sin1/1
  Gain9/1 -> Cos3/1
  Gain4/1 -> Cos1/1
  Cos2/1 -> Product3/1
  Product1/1 -> Mux1/2
  Gain7/1 -> Sin3/1
  Gain1/1 -> Sin/1
  Cos3/1 -> Product3/2
  R1/1 -> Gain4/1
  Y1/1 -> Gain5/1
  R2/1 -> Gain6/1
  Y2/1 -> Gain7/1
  Y3/1 -> Gain9/1
  R3/1 -> Gain8/1
  Y/1 -> Gain2/1
  R/1 -> Gain1/1
  Product2/1 -> Mux1/3

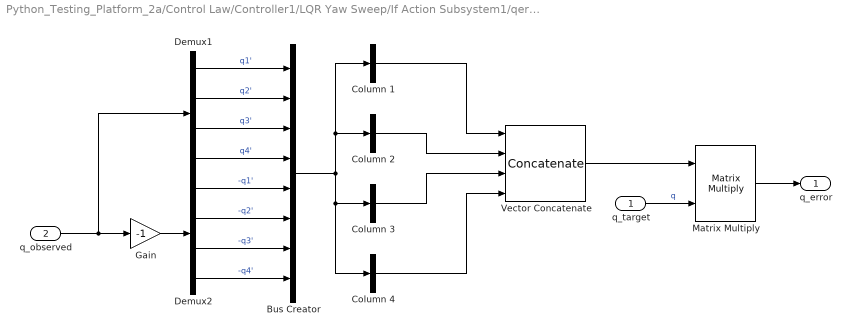
== system Python_Testing_Platform_2a/Control Law/Controller1/LQR Yaw Sweep/If Action Subsystem1/qerror/q ⦻ q' ==
  q_target : Inport
  q_observed : Inport  Port=2
  Bus Creator : BusCreator  Inputs=8
  Column 1 : BusSelector  OutputSignals=q4',-q3',q2',-q1'  OutputAsBus=on
  Column 2 : BusSelector  OutputSignals=q3',q4',-q1',-q2'  OutputAsBus=on
  Column 3 : BusSelector  OutputSignals=-q2',q1',q4',-q3'  OutputAsBus=on
  Column 4 : BusSelector  OutputSignals=q1',q2',q3',q4'  OutputAsBus=on
  Demux1 : Demux
  Demux2 : Demux
  Gain : Gain  Gain=-1
  Matrix Multiply : Product  Multiplication=Matrix(*)
  Vector Concatenate : Concatenate  NumInputs=4  Mode=Multidimensional array  ConcatenateDimension=2
  q_error : Outport
  wires:
  Gain/1 -> Demux2/1
  Demux1/1 -> Bus Creator/1  "q1'"
  Demux1/3 -> Bus Creator/3  "q3'"
  Demux1/2 -> Bus Creator/2  "q2'"
  Demux2/4 -> Bus Creator/8  "-q4'"
  Demux2/3 -> Bus Creator/7  "-q3'"
  Demux2/2 -> Bus Creator/6  "-q2'"
  Demux2/1 -> Bus Creator/5  "-q1'"
  Demux1/4 -> Bus Creator/4  "q4'"
  Bus Creator/1 -> Column 4/1, Column 3/1, Column 1/1, Column 2/1
  Column 1/1 -> Vector Concatenate/1
  Column 2/1 -> Vector Concatenate/2
  Column 3/1 -> Vector Concatenate/3
  Column 4/1 -> Vector Concatenate/4
  q_observed/1 -> Demux1/1, Gain/1
  q_target/1 -> Matrix Multiply/2  "q"
  Matrix Multiply/1 -> q_error/1
  Vector Concatenate/1 -> Matrix Multiply/1
